simulink model "motioncontrol"  (R2019b)
settings: Solver=VariableStepAuto  StartTime=0.0  StopTime=t_d  RelTol=1e-3
values from neighbouring files (symbols this model uses):
  a = [1;1]    [combined.m]    (also in forward.m = [1,1,1,1])
  F_v = K_r*diag([0.01 0.01])*K_r    [combined.m]
  g = 9.81    [combined.m]
  K_d = 750*diag([1 1])    [combined.m]
  K_p = 3750*diag([1 1])    [combined.m]
  pi_l = pi_m    [combined.m]
  q_i = x_d - 0.1    [combined.m]
  Tc = 0.001    [combined.m]
  Ts = Tc    (= 0.001)    [combined.m]
  x_d_dot = [1;5]    [combined.m]
  x_d_dot_dot = [2;5]    [combined.m]
undefined symbols (not defined in the file or in its folder): forward, iner_l, jac
settings Model: Creator=Administrator  LastModifiedBy=Administrator

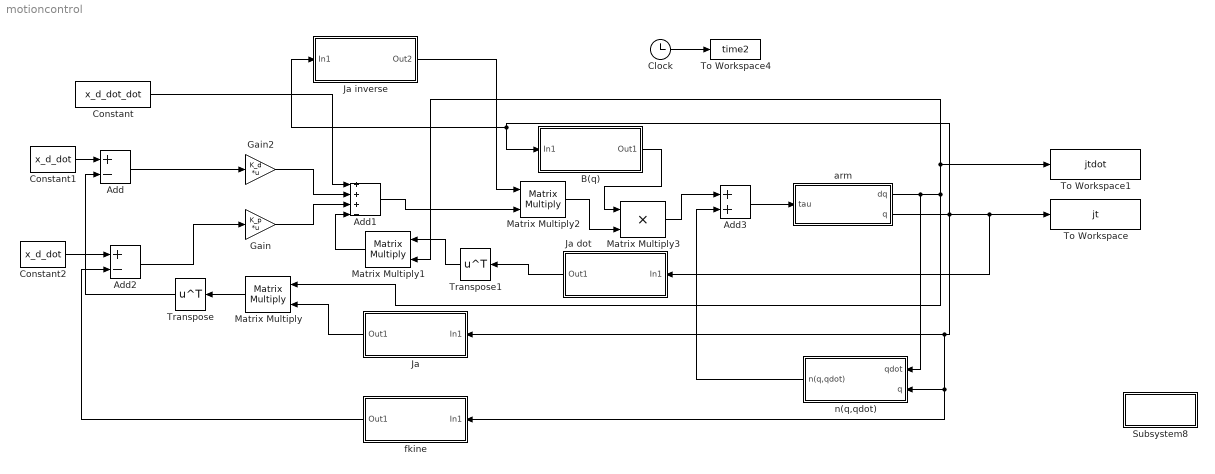
== system motioncontrol ==
  Add : Sum  Inputs=+-
  Add1 : Sum  Inputs=+++-
  Add2 : Sum  Inputs=+-
  Add3 : Sum
  B(q) : Subsystem
  Clock : Clock
  Constant : Constant  Value=x_d_dot_dot
  Constant1 : Constant  Value=x_d_dot
  Constant2 : Constant  Value=x_d_dot
  Gain : Gain  Gain=K_p  Multiplication=Matrix(K*u)  SampleTime=Tc
      mask Display: disp('K_p')
  Gain2 : Gain  Gain=K_d  Multiplication=Matrix(K*u)  SampleTime=Tc
      mask Display: disp('K_d')
  "Ja " : Subsystem
  Ja dot : Subsystem
  Ja inverse : Subsystem
  Matrix Multiply : Product  Multiplication=Matrix(*)
  Matrix Multiply1 : Product  Multiplication=Matrix(*)
  Matrix Multiply2 : Product  Multiplication=Matrix(*)
  Matrix Multiply3 : Product
  Subsystem8 : Subsystem
      settings: OpenFcn=p8_10;
      mask Display: disp('plot')
  To Workspace : ToWorkspace  VariableName=jt  SampleTime=Ts
      settings: MaxDataPoints=4001
  To Workspace1 : ToWorkspace  VariableName=jtdot  SampleTime=Ts
      settings: MaxDataPoints=4001
  To Workspace4 : ToWorkspace  VariableName=time2  SampleTime=Ts
      settings: MaxDataPoints=4001
  Transpose : Math  Operator=transpose  SignedPower=off  SaturateOnIntegerOverflow=on
  Transpose1 : Math  Operator=transpose  SignedPower=off  SaturateOnIntegerOverflow=on
  arm : Subsystem
      mask Display: disp('inv(B(q))(tau-tau'')')
  fkine : Subsystem
  n(q,qdot) : Subsystem
  wires:
  Add/1 -> Gain2/1
  Gain2/1 -> Add1/2
  Gain/1 -> Add1/3
  Constant1/1 -> Add/1
  Constant/1 -> Add1/1
  fkine/1(Out1) -> Add2/2
  Add2/1 -> Gain/1
  Add3/1 -> arm/1(tau)
  n(q,qdot)/1(n(q,qdot)) -> Add3/2
  Matrix Multiply2/1 -> Matrix Multiply3/2
  Matrix Multiply3/1 -> Add3/1
  Constant2/1 -> Add2/1
  Matrix Multiply1/1 -> Add1/4
  arm/1(dq) -> Matrix Multiply/1, To Workspace1/1, Matrix Multiply1/2, n(q,qdot)/1(qdot)
  arm/2("q ") -> To Workspace/1, Ja dot/1(In1), Ja inverse/1(In1), B(q)/1(In1), "Ja "/1(In1), fkine/1(In1), n(q,qdot)/2(q)
  Clock/1 -> To Workspace4/1
  "Ja "/1(Out1) -> Matrix Multiply/2
  Matrix Multiply/1 -> Transpose/1
  Transpose/1 -> Add/2
  Ja dot/1(Out1) -> Transpose1/1
  Transpose1/1 -> Matrix Multiply1/1
  B(q)/1(Out1) -> Matrix Multiply3/1
  Add1/1 -> Matrix Multiply2/2
  Ja inverse/1(Out2) -> Matrix Multiply2/1

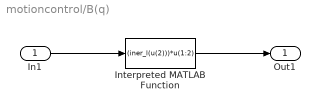
== system motioncontrol/B(q) ==
  In1 : Inport
  Interpreted MATLAB Function : MATLABFcn  MATLABFcn=(iner_l(u(2)))*u(1:2)  OutputDimensions=2
  Out1 : Outport
  wires:
  In1/1 -> Interpreted MATLAB Function/1
  Interpreted MATLAB Function/1 -> Out1/1

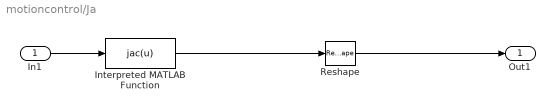
== system motioncontrol/Ja  ==
  In1 : Inport
  Interpreted MATLAB Function : MATLABFcn  MATLABFcn=jac(u)
  Reshape : Reshape  OutputDimensionality=Customize  OutputDimensions=[2,2]
  Out1 : Outport
  wires:
  Interpreted MATLAB Function/1 -> Reshape/1
  Reshape/1 -> Out1/1
  In1/1 -> Interpreted MATLAB Function/1

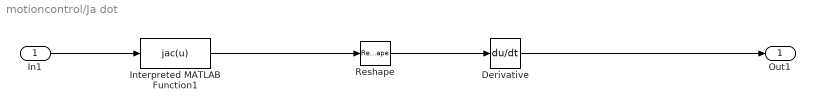
== system motioncontrol/Ja dot ==
  In1 : Inport
  Derivative : Derivative
  Interpreted MATLAB Function1 : MATLABFcn  MATLABFcn=jac(u)
  Reshape : Reshape  OutputDimensionality=Customize  OutputDimensions=[2,2]
  Out1 : Outport
  wires:
  Derivative/1 -> Out1/1
  In1/1 -> Interpreted MATLAB Function1/1
  Interpreted MATLAB Function1/1 -> Reshape/1
  Reshape/1 -> Derivative/1

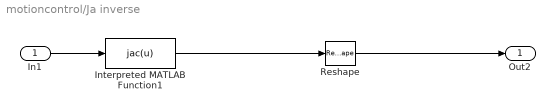
== system motioncontrol/Ja inverse ==
  In1 : Inport
  Interpreted MATLAB Function1 : MATLABFcn  MATLABFcn=jac(u)
  Reshape : Reshape  OutputDimensionality=Customize  OutputDimensions=[2,2]
  Out2 : Outport
  wires:
  In1/1 -> Interpreted MATLAB Function1/1
  Reshape/1 -> Out2/1
  Interpreted MATLAB Function1/1 -> Reshape/1

== system motioncontrol/Subsystem8 ==
  note: start

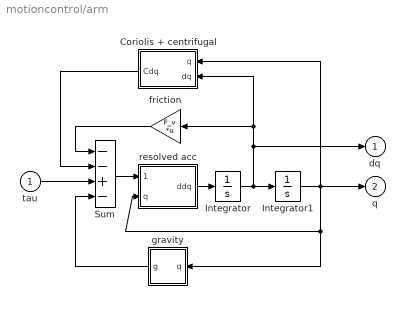
== system motioncontrol/arm ==
  tau : Inport
  Coriolis + centrifugal : Subsystem
      mask Display: disp('C(q,dq)dq')
  Integrator : Integrator  InitialCondition=[0 0]  ZeroCross=off
  Integrator1 : Integrator  InitialCondition=q_i  ZeroCross=off
  Sum : Sum  Inputs=--+-  SaturateOnIntegerOverflow=on  InputSameDT=on  OutDataTypeStr=Inherit: Same as first input
  friction : Gain  Gain=F_v  Multiplication=Matrix(K*u)  SaturateOnIntegerOverflow=on  OutDataTypeStr=Inherit: Same as input  ParamDataTypeStr=Inherit: Same as input
      mask Display: disp('F_v')
  gravity : Subsystem
      mask Display: disp('g(q)')
  resolved acc : Subsystem
      mask Display: disp('inv(B(q))')
  dq : Outport  InitialOutput=0
  "q " : Outport  Port=2  InitialOutput=0
  wires:
  Coriolis + centrifugal/1(Cdq) -> Sum/2
  tau/1 -> Sum/3
  Integrator1/1 -> Coriolis + centrifugal/1(q), resolved acc/2(q), gravity/1(q), "q "/1
  resolved acc/1(ddq) -> Integrator/1
  Integrator/1 -> Integrator1/1, dq/1, Coriolis + centrifugal/2(dq), friction/1
  Sum/1 -> resolved acc/1(tau-tau')
  friction/1 -> Sum/1
  gravity/1(g) -> Sum/4

== system motioncontrol/fkine ==
  In1 : Inport
  Interpreted MATLAB Function : MATLABFcn  MATLABFcn=forward(u)
  Out1 : Outport
  wires:
  In1/1 -> Interpreted MATLAB Function/1
  Interpreted MATLAB Function/1 -> Out1/1

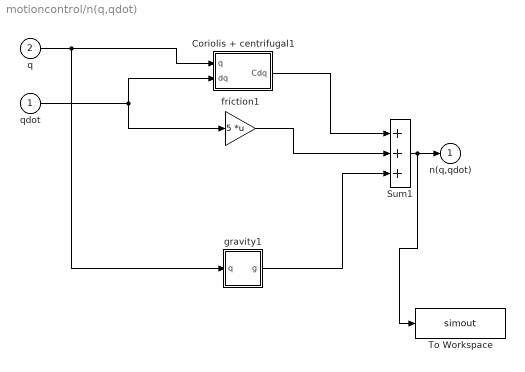
== system motioncontrol/n(q,qdot) ==
  qdot : Inport
  q : Inport  Port=2
  Coriolis + centrifugal1 : Subsystem
      mask Display: disp('C(q,dq)dq')
  Sum1 : Sum  Inputs=+++  SaturateOnIntegerOverflow=on  InputSameDT=on  OutDataTypeStr=Inherit: Same as first input
  To Workspace : ToWorkspace  VariableName=simout  SaveFormat=Timeseries  SampleTime=-1
  friction1 : Gain  Gain=5  Multiplication=Matrix(K*u)  SaturateOnIntegerOverflow=on  OutDataTypeStr=Inherit: Same as input  ParamDataTypeStr=Inherit: Same as input
      mask Display: disp('F_v')
  gravity1 : Subsystem
      mask Display: disp('g(q)')
  n(q,qdot) : Outport  InitialOutput=0
  wires:
  q/1 -> gravity1/1(q), Coriolis + centrifugal1/1(q)
  Coriolis + centrifugal1/1(Cdq) -> Sum1/1
  ? -> ?
  friction1/1 -> Sum1/2
  Sum1/1 -> To Workspace/1, n(q,qdot)/1
  qdot/1 -> friction1/1, Coriolis + centrifugal1/2(dq)
  gravity1/1(g) -> Sum1/3

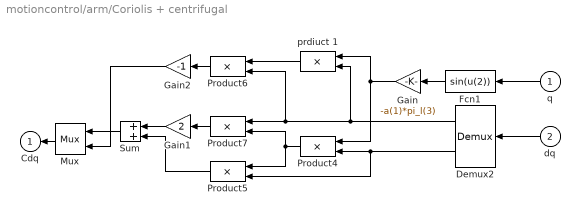
== system motioncontrol/arm/Coriolis + centrifugal ==
  q : Inport
  dq : Inport  Port=2
  Demux2 : Demux  Outputs=2
  Fcn1 : Fcn  Expr=sin(u(2))
  Gain : Gain  Gain=-a(1)*pi_l(3)  SaturateOnIntegerOverflow=on  OutDataTypeStr=Inherit: Same as input  ParamDataTypeStr=Inherit: Same as input
      mask Display: disp('k_3')
  Gain1 : Gain  Gain=2  SaturateOnIntegerOverflow=on  OutDataTypeStr=Inherit: Same as input  ParamDataTypeStr=Inherit: Same as input
  Gain2 : Gain  Gain=-1  SaturateOnIntegerOverflow=on  OutDataTypeStr=Inherit: Same as input  ParamDataTypeStr=Inherit: Same as input
  Mux : Mux  Inputs=2
  Product{4..7} (4 alike) : Product  SaturateOnIntegerOverflow=on  RndMeth=Zero  InputSameDT=on  OutDataTypeStr=Inherit: Same as first input
  Sum : Sum  SaturateOnIntegerOverflow=on  InputSameDT=on  OutDataTypeStr=Inherit: Same as first input
  prdiuct 1 : Product  SaturateOnIntegerOverflow=on  RndMeth=Zero  InputSameDT=on  OutDataTypeStr=Inherit: Same as first input
  Cdq : Outport  InitialOutput=0
  wires:
  dq/1 -> Demux2/1
  Gain2/1 -> Mux/2
  Product6/1 -> Gain2/1
  Mux/1 -> Cdq/1
  Sum/1 -> Mux/1
  Product5/1 -> Sum/2
  Gain1/1 -> Sum/1
  Product7/1 -> Gain1/1
  Demux2/1 -> prdiuct 1/2, Product6/2, Product7/1
  Demux2/2 -> Product4/2, Product5/2
  prdiuct 1/1 -> Product6/1
  Gain/1 -> prdiuct 1/1, Product4/1
  Fcn1/1 -> Gain/1
  q/1 -> Fcn1/1
  Product4/1 -> Product5/1, Product7/2

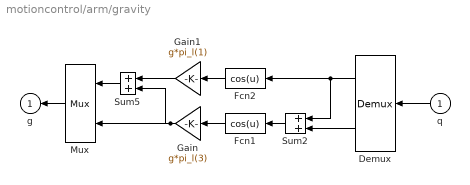
== system motioncontrol/arm/gravity ==
  q : Inport
  Demux : Demux  Outputs=2
  Fcn1 : Fcn  Expr=cos(u)
  Fcn2 : Fcn  Expr=cos(u)
  Gain : Gain  Gain=g*pi_l(3)  SaturateOnIntegerOverflow=on  OutDataTypeStr=Inherit: Same as input  ParamDataTypeStr=Inherit: Same as input
      mask Display: disp('k_2')
  Gain1 : Gain  Gain=g*pi_l(1)  SaturateOnIntegerOverflow=on  OutDataTypeStr=Inherit: Same as input  ParamDataTypeStr=Inherit: Same as input
      mask Display: disp('k_1')
  Mux : Mux  Inputs=2
  Sum2 : Sum  SaturateOnIntegerOverflow=on  InputSameDT=on  OutDataTypeStr=Inherit: Same as first input
  Sum5 : Sum  SaturateOnIntegerOverflow=on  InputSameDT=on  OutDataTypeStr=Inherit: Same as first input
  g : Outport  InitialOutput=0
  wires:
  q/1 -> Demux/1
  Demux/2 -> Sum2/2
  Sum2/1 -> Fcn1/1
  Fcn1/1 -> Gain/1
  Fcn2/1 -> Gain1/1
  Demux/1 -> Fcn2/1, Sum2/1
  Gain1/1 -> Sum5/1
  Sum5/1 -> Mux/1
  Gain/1 -> Sum5/2, Mux/2
  Mux/1 -> g/1

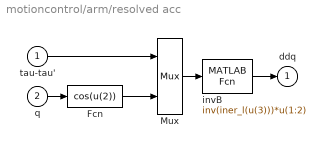
== system motioncontrol/arm/resolved acc ==
  tau-tau' : Inport
  q : Inport  Port=2
  Fcn : Fcn  Expr=cos(u(2))
  Mux : Mux  Inputs=[2,1]
  "invB " : MATLABFcn  MATLABFcn=inv(iner_l(u(3)))*u(1:2)  OutputDimensions=2
      mask Display: disp('inv(B(q))')
  ddq : Outport  InitialOutput=0
  wires:
  Fcn/1 -> Mux/2
  q/1 -> Fcn/1
  "invB "/1 -> ddq/1
  tau-tau'/1 -> Mux/1
  Mux/1 -> "invB "/1

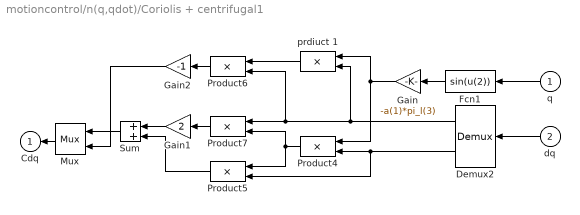
== system motioncontrol/n(q,qdot)/Coriolis + centrifugal1 ==
  q : Inport
  dq : Inport  Port=2
  Demux2 : Demux  Outputs=2
  Fcn1 : Fcn  Expr=sin(u(2))
  Gain : Gain  Gain=-a(1)*pi_l(3)  SaturateOnIntegerOverflow=on  OutDataTypeStr=Inherit: Same as input  ParamDataTypeStr=Inherit: Same as input
      mask Display: disp('k_3')
  Gain1 : Gain  Gain=2  SaturateOnIntegerOverflow=on  OutDataTypeStr=Inherit: Same as input  ParamDataTypeStr=Inherit: Same as input
  Gain2 : Gain  Gain=-1  SaturateOnIntegerOverflow=on  OutDataTypeStr=Inherit: Same as input  ParamDataTypeStr=Inherit: Same as input
  Mux : Mux  Inputs=2
  Product{4..7} (4 alike) : Product  SaturateOnIntegerOverflow=on  RndMeth=Zero  InputSameDT=on  OutDataTypeStr=Inherit: Same as first input
  Sum : Sum  SaturateOnIntegerOverflow=on  InputSameDT=on  OutDataTypeStr=Inherit: Same as first input
  prdiuct 1 : Product  SaturateOnIntegerOverflow=on  RndMeth=Zero  InputSameDT=on  OutDataTypeStr=Inherit: Same as first input
  Cdq : Outport  InitialOutput=0
  wires:
  dq/1 -> Demux2/1
  Gain2/1 -> Mux/2
  Product6/1 -> Gain2/1
  Mux/1 -> Cdq/1
  Sum/1 -> Mux/1
  Product5/1 -> Sum/2
  Gain1/1 -> Sum/1
  Product7/1 -> Gain1/1
  Demux2/1 -> prdiuct 1/2, Product6/2, Product7/1
  Demux2/2 -> Product4/2, Product5/2
  prdiuct 1/1 -> Product6/1
  Gain/1 -> prdiuct 1/1, Product4/1
  Fcn1/1 -> Gain/1
  q/1 -> Fcn1/1
  Product4/1 -> Product5/1, Product7/2

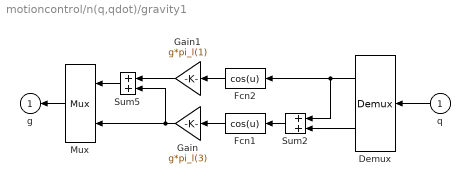
== system motioncontrol/n(q,qdot)/gravity1 ==
  q : Inport
  Demux : Demux  Outputs=2
  Fcn1 : Fcn  Expr=cos(u)
  Fcn2 : Fcn  Expr=cos(u)
  Gain : Gain  Gain=g*pi_l(3)  SaturateOnIntegerOverflow=on  OutDataTypeStr=Inherit: Same as input  ParamDataTypeStr=Inherit: Same as input
      mask Display: disp('k_2')
  Gain1 : Gain  Gain=g*pi_l(1)  SaturateOnIntegerOverflow=on  OutDataTypeStr=Inherit: Same as input  ParamDataTypeStr=Inherit: Same as input
      mask Display: disp('k_1')
  Mux : Mux  Inputs=2
  Sum2 : Sum  SaturateOnIntegerOverflow=on  InputSameDT=on  OutDataTypeStr=Inherit: Same as first input
  Sum5 : Sum  SaturateOnIntegerOverflow=on  InputSameDT=on  OutDataTypeStr=Inherit: Same as first input
  g : Outport  InitialOutput=0
  wires:
  q/1 -> Demux/1
  Demux/2 -> Sum2/2
  Sum2/1 -> Fcn1/1
  Fcn1/1 -> Gain/1
  Fcn2/1 -> Gain1/1
  Demux/1 -> Fcn2/1, Sum2/1
  Gain1/1 -> Sum5/1
  Sum5/1 -> Mux/1
  Gain/1 -> Sum5/2, Mux/2
  Mux/1 -> g/1
